simulink model "tf_light_contr"  (R2020a)
settings: Solver=FixedStepDiscrete  StartTime=0.0  StopTime=inf  FixedStep=0.001  RelTol=1e-3
settings Model: NumberOfSteps=5000  Creator=deepak  LastModifiedBy=deepak

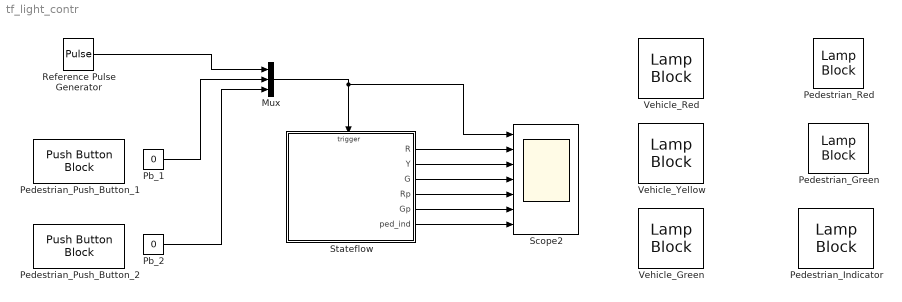
== system tf_light_contr ==
  Mux : Mux  Inputs=3
  Pb_1 : Constant  Value=0
  Pb_2 : Constant  Value=0
  Pedestrian_Green : LampBlock
  Pedestrian_Indicator : LampBlock
  Pedestrian_Push_Button_1 : PushButtonBlock  LabelPosition=Top
  Pedestrian_Push_Button_2 : PushButtonBlock  LabelPosition=Top
  Pedestrian_Red : LampBlock
  Reference Pulse Generator : DiscretePulseGenerator  PulseType=Time based  Period=10  PulseWidth=50  SampleTime=0.1
  Scope2 : Scope  NumInputPorts=7
  Stateflow : Stateflow chart  TreatAsAtomicUnit=on
  Vehicle_Green : LampBlock
  Vehicle_Red : LampBlock
  Vehicle_Yellow : LampBlock
  wires:
  Stateflow/1(R) -> Scope2/2
  Reference Pulse Generator/1 -> Mux/1
  Stateflow/5(Gp) -> Scope2/6
  Stateflow/4(Rp) -> Scope2/5
  Stateflow/3(G) -> Scope2/4
  Stateflow/2(Y) -> Scope2/3
  Mux/1 -> Stateflow/Trigger, Scope2/1
  Pb_1/1 -> Mux/2
  Stateflow/6(ped_ind) -> Scope2/7
  Pb_2/1 -> Mux/3

== stateflow chart tf_light_contr/Stateflow ==
  settings: executeAtInitialization=1
  state Default_state
    en: R = 0;
    Y = 0;
    G = 1;
    Rp = 1;
    Gp = 0;
    ped_ind = 0;
  state Activate_Ped_cross
    state Road [parallel]
      settings: executionOrder=1
      state Go
        en: R = 0;
        Y = 0;
        G = 1;
        Rp = 1;
        Gp = 0;
        N = timer_G;
        ped_ind = 1;
      state Caution_Stop
        en: R = 0;
        Y = 1;
        G = 0;
        Rp = 1;
        Gp = 0;
        N = timer_Y;
        ped_ind = 1;
      state Stop
        en: R = 1;
        Y = 0;
        G = 0;
        Rp = 0;
        Gp = 1;
        N = timer_R;
        ped_ind = 0;
      state Caution_Go
        en: R = 1;
        Y = 1;
        G = 0;
        Rp = 1;
        Gp = 0;
        N = timer_RY;
        ped_ind = 0;
      (default) -> Go
      Go -> Caution_Stop : [nx_state == 1]
      Caution_Stop -> Stop : [nx_state == 1]
      Stop -> Caution_Go : [nx_state == 1]
    state Clock_signal [parallel]
      settings: executionOrder=2
      state clk_count_check(cnt) [function]
        (default) -> (junction 72) : % clk_count
        (junction 72) -> (junction 73) [order 1] : [cnt == N]
        (junction 72) -> (junction 74) [order 2] : {nx_state = 0 }
        (junction 73) -> (junction 75) : {nx_state = 1, count = 0;}
        (junction 75) -> (junction 74)
        (junction 74) -> (junction 76)
      state Clock
        en: clk_count_check(count)
      (default) -> Clock
      Clock -> Clock : [clk]{count = count + 1}
  (default) -> Default_state
  Caution_Go -> Default_state : [nx_state == 1]
  Default_state -> Activate_Ped_cross : [req_1 | req_2 ]
  data: cnt function_input double; R output; Y output; G output; N local =1; Rp output; Gp output; count local double =0; nx_state local; ped_ind output; timer_G constant double =20; timer_Y constant double =15; timer_R constant double =20; timer_RY constant double =15
  events: clk input RISING_EDGE_EVENT; req_1 input FALLING_EDGE_EVENT; req_2 input FALLING_EDGE_EVENT
